simulink model "adaptive_cruise_control_v2"  (R2019a)
settings: Solver=FixedStepAuto  StartTime=0.0  StopTime=inf  RelTol=1e-3  EnableMultiTasking=on
libraries: arduinolib x5, LCDlib x1, arduinosensorlib x1
settings Model: SimulationMode=external  ExtModeTrigDuration=2  Creator=Shyam lal  LastModifiedBy=phani
settings OptimizationCC: EnhancedBackFolding=on  PassReuseOutputArgsAs=Individual arguments  MaxStackSize=64  OptimizeBlockOrder=speed  DifferentSizesBufferReuse=on  OptimizationCustomize=off
settings DebuggingCC: ParameterTunabilityLossMsg=error
settings HardwareCC: ProdBitPerInt=16  ProdBitPerPointer=16  ProdBitPerSizeT=16  ProdBitPerPtrDiffT=16  ProdLargestAtomicFloat=None  ProdWordSize=8  ProdHWDeviceType=Atmel->AVR
settings SFSimCC: MATLABDynamicMemAlloc=off
settings RTWCC: SystemTargetFile=ert.tlc  HardwareBoard=Arduino Uno  TLCOptions=-aInlineSetEventsForThisBaseRateFcn=TLC_FALSE -aSuppressMultiTaskScheduler=TLC_FALSE -aRateBasedStepFcn=1  TemplateMakefile=ert_default_tmf  GenerateReport=on  Toolchain=Arduino AVR  BuildConfiguration=Faster Runs  IncludeHyperlinkInReport=on  LaunchReport=on  GenerateTraceInfo=on  GenerateTraceReport=on  GenerateTraceReportSl=on  GenerateTraceReportSf=on  GenerateTraceReportEml=on
settings CodeAppCC: ForceParamTrailComments=on  IgnoreCustomStorageClasses=off  OperatorAnnotations=on  SimulinkDataObjDesc=on  SFDataObjDesc=on  InsertBlockDesc=on
settings ERTTargetCC: SupportContinuousTime=on  SupportVariableSizeSignals=on  ExtModeStaticAllocSize=250

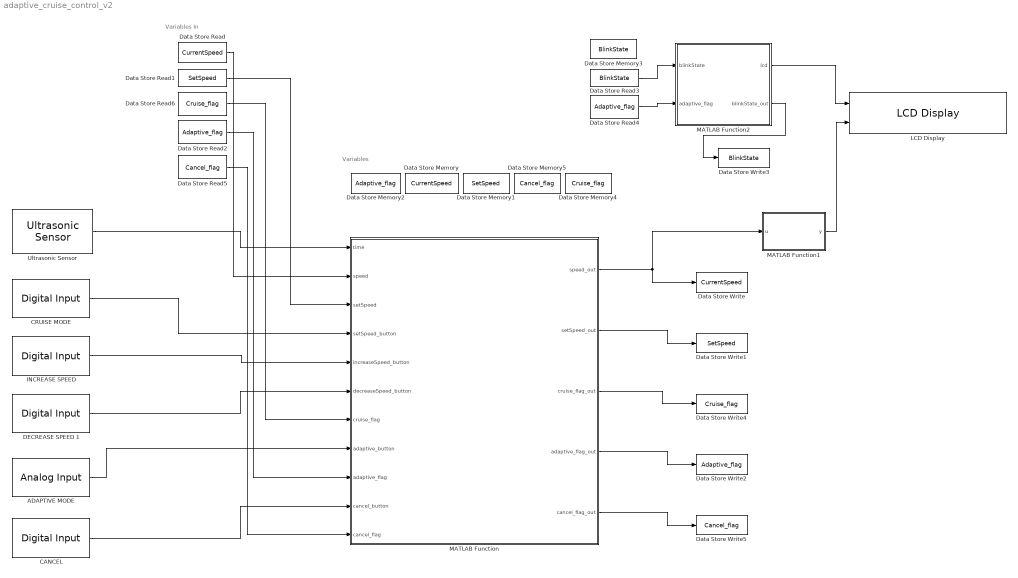
== system adaptive_cruise_control_v2 ==
  note: Variables
  note: Variables In
  ADAPTIVE MODE : arduinolib/Analog Input  pinNumber=3  ReadResultsOnly=off  ConversionTriggerSource=Software  ExternalTriggerType=uint32(0)  OutputDataType=uint16  EnableConversionCompleteNotify=off  EnableOuputStatus=off  SampleTime=.5  blockPlatform=arduino
  "CANCEL " : arduinolib/Digital Input  pinNumber=5  sampleTime=.5  blockPlatform=arduino
      settings: SourceProductName=Simulink Support Package for Arduino Hardware
  CRUISE MODE : arduinolib/Digital Input  pinNumber=4  sampleTime=.5  blockPlatform=arduino
      settings: SourceProductName=Simulink Support Package for Arduino Hardware
  DECREASE SPEED 1 : arduinolib/Digital Input  pinNumber=13  sampleTime=.5  blockPlatform=arduino
      settings: SourceProductName=Simulink Support Package for Arduino Hardware
  Data Store Memory : DataStoreMemory  DataStoreName=CurrentSpeed  ReadBeforeWriteMsg=warning  WriteAfterWriteMsg=warning  WriteAfterReadMsg=warning  ShowAdditionalParam=off
  Data Store Memory1 : DataStoreMemory  DataStoreName=SetSpeed  ReadBeforeWriteMsg=warning  WriteAfterWriteMsg=warning  WriteAfterReadMsg=warning  ShowAdditionalParam=off
  Data Store Memory2 : DataStoreMemory  DataStoreName=Adaptive_flag  ReadBeforeWriteMsg=warning  WriteAfterWriteMsg=warning  WriteAfterReadMsg=warning  ShowAdditionalParam=off
  Data Store Memory3 : DataStoreMemory  DataStoreName=BlinkState  ReadBeforeWriteMsg=warning  WriteAfterWriteMsg=warning  WriteAfterReadMsg=warning  ShowAdditionalParam=off
  Data Store Memory4 : DataStoreMemory  DataStoreName=Cruise_flag  ReadBeforeWriteMsg=warning  WriteAfterWriteMsg=warning  WriteAfterReadMsg=warning  ShowAdditionalParam=off
  Data Store Memory5 : DataStoreMemory  DataStoreName=Cancel_flag  ReadBeforeWriteMsg=warning  WriteAfterWriteMsg=warning  WriteAfterReadMsg=warning  ShowAdditionalParam=off
  Data Store Read : DataStoreRead  DataStoreName=CurrentSpeed
  Data Store Read1 : DataStoreRead  DataStoreName=SetSpeed
  Data Store Read2 : DataStoreRead  DataStoreName=Adaptive_flag
  Data Store Read3 : DataStoreRead  DataStoreName=BlinkState
  Data Store Read4 : DataStoreRead  DataStoreName=Adaptive_flag
  Data Store Read5 : DataStoreRead  DataStoreName=Cancel_flag
  Data Store Read6 : DataStoreRead  DataStoreName=Cruise_flag
  Data Store Write : DataStoreWrite  DataStoreName=CurrentSpeed
  Data Store Write1 : DataStoreWrite  DataStoreName=SetSpeed
  Data Store Write2 : DataStoreWrite  DataStoreName=Adaptive_flag
  Data Store Write3 : DataStoreWrite  DataStoreName=BlinkState
  Data Store Write4 : DataStoreWrite  DataStoreName=Cruise_flag
  Data Store Write5 : DataStoreWrite  DataStoreName=Cancel_flag
  "INCREASE SPEED " : arduinolib/Digital Input  pinNumber=12  sampleTime=.5  blockPlatform=arduino
      settings: SourceProductName=Simulink Support Package for Arduino Hardware
  LCD Display : LCDlib/LCD Display  pins=[6,7,8,9,10,11]
      settings: SourceProductName=LCD Library
  MATLAB Function : MATLAB Function  TreatAsAtomicUnit=on
  MATLAB Function1 : MATLAB Function  TreatAsAtomicUnit=on
  MATLAB Function2 : MATLAB Function  TreatAsAtomicUnit=on
  Ultrasonic Sensor : arduinosensorlib/Ultrasonic Sensor  NumSignalPins=2  TrigPin=2  EchoPin=3  SignalPin=3  SampleTime_=.5  blockPlatform=ARDUINO
      settings: SourceProductName=Simulink Support Package for Arduino Hardware  SourceProductBaseCode=ARDUINO
  wires:
  MATLAB Function/1(speed_out) -> MATLAB Function1/1(u), Data Store Write/1
  MATLAB Function2/2(blinkState_out) -> Data Store Write3/1
  MATLAB Function1/1(y) -> LCD Display/2
  MATLAB Function2/1(lcd) -> LCD Display/1
  Data Store Read4/1 -> MATLAB Function2/2(adaptive_flag)
  Data Store Read3/1 -> MATLAB Function2/1(blinkState)
  MATLAB Function/5(cancel_flag_out) -> Data Store Write5/1
  MATLAB Function/4(adaptive_flag_out) -> Data Store Write2/1
  MATLAB Function/3(cruise_flag_out) -> Data Store Write4/1
  MATLAB Function/2(setSpeed_out) -> Data Store Write1/1
  "CANCEL "/1 -> MATLAB Function/10(cancel_button)
  "INCREASE SPEED "/1 -> MATLAB Function/5(increaseSpeed_button)
  CRUISE MODE/1 -> MATLAB Function/4(setSpeed_button)
  DECREASE SPEED 1/1 -> MATLAB Function/6(decreaseSpeed_button)
  Data Store Read6/1 -> MATLAB Function/7(cruise_flag)
  Data Store Read2/1 -> MATLAB Function/9(adaptive_flag)
  Data Store Read/1 -> MATLAB Function/2(speed)
  Data Store Read1/1 -> MATLAB Function/3(setSpeed)
  Ultrasonic Sensor/1 -> MATLAB Function/1(time)
  Data Store Read5/1 -> MATLAB Function/11(cancel_flag)
  ADAPTIVE MODE/1 -> MATLAB Function/8(adaptive_button)

== matlab function adaptive_cruise_control_v2/MATLAB Function1 ==
  data: y output; u input
function y = fcn_test(u)
switch u
    case 0
        y = [[48],[48]];
    case 1
        y = [[48],[49]];
    case 2 
        y = [[48],[50]];
    case 3
        y = [[48],[51]];
    case 4
        y = [[48],[52]];
    case 5
        y = [[48],[53]];
    case 6
        y = [[48],[54]];
    case 7
        y = [[48],[55]];
    case 8
        y = [[48],[56]];
    case 9
        y = [[48],[57]];
    case 10
        y = [[49],[48]];
    case 11 
        y = [[49],[49]];
    case 12
        y = [[49],[50]];
    case 13
        y = [[49],[51]];
    case 14
        y = [[49],[52]];
    case 15
        y = [[49],[53]];
    case 16
        y = [[49],[54]];
    case 17
        y = [[49],[55]];
    case 18
        y = [[49],[56]];
    case 19
        y = [[49],[57]];
    case 20
        y = [[50],[48]];
    case 21 
        y = [[50],[49]];
    case 22
        y = [[50],[50]];
    case 23
        y = [[50],[51]];
    case 24
        y = [[50],[52]];
    case 25
        y = [[50],[53]];
    case 26
        y = [[50],[54]];
    case 27
        y = [[50],[55]];
    case 28
        y = [[50],[56]];
    case 29
        y = [[50],[57]];
    case 30
        y = [[51],[48]];
    case 31 
        y = [[51],[49]];
    case 32
        y = [[51],[50]];
    case 33
        y = [[51],[51]];
    case 34
        y = [[51],[52]];
    case 35
        y = [[51],[53]];
    case 36
        y = [[51],[54]];
    case 37
        y = [[51],[55]];
    case 38
        y = [[51],[56]];
    case 39
        y = [[51],[57]];
    case 40
        y = [[52],[48]];
    case 41 
        y = [[52],[49]];
    case 42
        y = [[52],[50]];
    case 43
        y = [[52],[51]];
    case 44
        y = [[52],[52]];
    case 45
        y = [[52],[53]];
    case 46
        y = [[52],[54]];
    case 47
        y = [[52],[55]];
    case 48
        y = [[52],[56]];
    case 49
        y = [[52],[57]];
    case 50
        y = [[53],[48]];
    case 51 
        y = [[53],[49]];
    case 52
        y = [[53],[50]];
    case 53
        y = [[53],[51]];
    case 54
        y = [[53],[52]];
    case 55
        y = [[53],[53]];
    case 56
        y = [[53],[54]];
    case 57
        y = [[53],[55]];
    case 58
        y = [[53],[56]];
    case 59
        y = [[53],[57]];
    case 60
        y = [[54],[48]];
    case 61 
        y = [[54],[49]];
    case 62
        y = [[54],[50]];
    case 63
        y = [[54],[51]];
    case 64
        y = [[54],[52]];
    case 65
        y = [[54],[53]];
    case 66
        y = [[54],[54]];
    case 67
        y = [[54],[55]];
    case 68
        y = [[54],[56]];
    case 69
        y = [[54],[57]];
    case 70
        y = [[55],[48]];
    case 71 
        y = [[55],[49]];
    case 72
        y = [[55],[50]];
    case 73
        y = [[55],[51]];
    case 74
        y = [[55],[52]];
    case 75
        y = [[55],[53]];
    case 76
        y = [[55],[54]];
    case 77
        y = [[55],[55]];
    case 78
        y = [[55],[56]];
    case 79
        y = [[55],[57]];
    case 80
        y = [[56],[48]];
    case 81 
        y = [[56],[49]];
    case 82
        y = [[56],[50]];
    case 83
        y = [[56],[51]];
    case 84
        y = [[56],[52]];
    case 85
        y = [[56],[53]];
    case 86
        y = [[56],[54]];
    case 87
        y = [[56],[55]];
    case 88
        y = [[56],[56]];
    case 89
        y = [[56],[57]];
    case 90
        y = [[57],[48]];
    case 91 
        y = [[57],[49]];
    case 92
        y = [[57],[50]];
    case 93
        y = [[57],[51]];
    case 94
        y = [[57],[52]];
    case 95
        y = [[57],[53]];
    case 96
        y = [[57],[54]];
    case 97
        y = [[57],[55]];
    case 98
        y = [[57],[56]];
    case 99
        y = [[57],[57]];
    otherwise
        y = [[48],[48]];
end

== matlab function adaptive_cruise_control_v2/MATLAB Function ==
  data: time input; speed_out output; speed input; setSpeed input; setSpeed_button input; increaseSpeed_button input; decreaseSpeed_button input; cruise_flag input; setSpeed_out output; cruise_flag_out output; adaptive_button input; adaptive_flag input; adaptive_flag_out output; cancel_button input; cancel_flag input; cancel_flag_out output
% Program Adaptive_Cruise_Control.m:
% Adjusts the speed of a car based on the obstacle in front along with
% normal cruise mode(maintaining a constant speed)
% Created on Feb 22, 2020 by SHYAM LAL LAKSHMIRAMIYA SRIDHAR, JITEN
% RAJENDRA PANDIT,PHANI TEJASWINI KARNATI

% Input Variables:
% time = time taken for the ultrasonic waves to reach the receiver end of
% the ultrasonic sensor.
% speed = current speed of the vehicle.
% setSpeed = locked speed of the vehicle in cruise mode.
% setSpeed_button = input from cruise mode button.
% increaseSpeed_button = input from increase speed button.
% decreaseSpeed_button = input from decrease speed button.
% cruise_flag = flag to represent the vehicle in cruise mode.
% adaptive_button = input from the adaptive cruise button.
% adaptive_flag = flag to represent the vehicle in Adaptive Cruise mode.
% cancel_button = input from the cancel mode button
% cancel_flag = flag to represent the vehicle is not in any driving mode.

% Output Variables:
% speed_out = updated current speed of the vehicle.
% setSpeed_out = updated locked speed of the vehicle in cruise mode. 
% cruise_flag_out = updated flag to represent the vehicle in cruise mode.
% adaptive_flag_out = updated flag to represent the vehicle in Adaptive Cruise mode.
% cancel_flag_out = updated flag to represent the vehicle is not in any driving mode.

function [speed_out, setSpeed_out,cruise_flag_out, adaptive_flag_out, cancel_flag_out] = Adaptive_Cruise_Control(time,speed,setSpeed,setSpeed_button,increaseSpeed_button, decreaseSpeed_button,cruise_flag,adaptive_button,adaptive_flag,cancel_button,cancel_flag)
    % Calculating the distance of the obstacle in front of the ultrasonic sensor.
    distance=(time*343)/2;
    
    % Setting flags for different driving modes.
    if cancel_button % Checking cancel button input and resetting all other modes flags.
        cancel_flag_out=1;
        adaptive_flag_out=0;
        setSpeed_out=setSpeed;
        cruise_flag_out=0;
    elseif adaptive_button>600 % Checking adaptive button input and setting the adaptive cruise mode flags.
        setSpeed_out=speed;
        adaptive_flag_out=1;
        cancel_flag_out=0;
        cruise_flag_out=0;
    elseif setSpeed_button % Checking set button input and setting the normal cruise mode flags.
        setSpeed_out=speed; % Locking the current speed
        cruise_flag_out=1;
        cancel_flag_out=cancel_flag;
        adaptive_flag_out=0;
    else % Retaining flag values when not in any mode.
        setSpeed_out=setSpeed;
        cruise_flag_out=cruise_flag;
        adaptive_flag_out=adaptive_flag;
        cancel_flag_out=cancel_flag;
    end
    
    if increaseSpeed_button && ~adaptive_flag
        speed_out = speed+1; % Increasing Speed 
    elseif decreaseSpeed_button && speed>0 && ~adaptive_flag
        speed_out = speed-1; % Decreasing Speed 
    elseif cruise_flag % Cruise Mode
        if increaseSpeed_button && ~adaptive_flag % increase speed and lock.
            speed_out = speed+1;
            setSpeed_out = speed;
        elseif decreaseSpeed_button && speed>0 && ~adaptive_flag % decrease speed and lock.
            speed_out = speed-1;
            setSpeed_out = speed;
        else
            speed_out = speed;
            setSpeed_out = setSpeed;
        end
    elseif adaptive_flag % Adaptive Cruise Mode
        if (distance<20) && (speed>0)
            speed_out=speed-2; % Decreasing speed by 2 if the obstacle is very near to the car.
        elseif (distance>=20) && (distance<30) && (speed>0)
            speed_out=speed-1; % Decreasing speed by 1 if the obstacle is near to the car.
        else % Bringing the speed to the set speed if no obstacle is found.
            if setSpeed<1
                speed_out=speed;
            else
                if speed<setSpeed
                    if distance<=30
                        speed_out=speed;
                    else
                        speed_out=speed+1;
                    end
                elseif speed>setSpeed && speed>0
                    speed_out=speed-1;
                else
                    speed_out=speed;
                end
            end
        end
    elseif cancel_flag || cancel_flag_out % Bring the current speed to 0.
        if speed>0
            speed_out=speed-1;
        else
            speed_out=speed;
            cancel_flag_out=0;
        end
    else % Bring the current speed to 0 if not in any mode.
        if speed>0
            speed_out=speed-1;
        else
            speed_out=speed;
        end
    end
end

== matlab function adaptive_cruise_control_v2/MATLAB Function2 ==
  data: lcd output; blinkState input; blinkState_out output; adaptive_flag input
% Program blinkFcn.m:
% Blink the LCD Display for differentiating ACC Mode.
% Created on Feb 22, 2020 by SHYAM LAL LAKSHMIRAMIYA SRIDHAR, JITEN
% RAJENDRA PANDIT,PHANI TEJASWINI KARNATI

% Input Variables:
% blinkState = flag to represent the blinking toggle value.
% adaptive_flag = flag to represent the vehicle in Adaptive Cruise mode.

% Output Variables:
% lcd = input to the Line 2 of LCD Display.
% blinkState_out = update flag to represent the blinking toggle value.
function [lcd,blinkState_out]  = blinkFcn(blinkState,adaptive_flag)

    if blinkState==0 && adaptive_flag
        lcd=[[32],[32],[32],[32],[32],[32]];
        blinkState_out=1;
    elseif blinkState==1 && adaptive_flag
        lcd=[[83],[112],[101],[101],[100],[58]]; 
        blinkState_out=0;
    else
        lcd=[[83],[112],[101],[101],[100],[58]];
        blinkState_out=blinkState;
    end
end
